simulink model "inga2s"  (R2013a)
settings: Solver=ode45  StartTime=0.0  StopTime=100.0  RelTol=1e-3
values from neighbouring files (symbols this model uses):
  b = 0.3    [Inga.m]
  g = 9.81    [Inga.m]
  J = 0.008    [Inga.m]
  l = 6    [Inga.m]
  m = 0.4    [Inga.m]
  M = 0.6    [Inga.m]
settings Model: Creator=Kinga  LastModifiedBy=rudi
settings DataIOCC: SignalLoggingSaveFormat=ModelDataLogs
settings DebuggingCC: UnderspecifiedInitializationDetection=Simplified  MultiTaskDSMMsg=warning  MultiTaskCondExecSysMsg=none  StateNameClashWarn=none  StrictBusMsg=ErrorOnBusTreatedAsVector  NonBusSignalsTreatedAsBus=error
settings RTWCC: IncludeERTFirstTime=on
settings GRTTargetCC: CodeReplacementLibrary=None  CPPClassGenCompliant=on

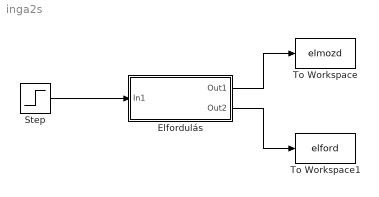
== system inga2s ==
  Elfordulás : Subsystem
  Step : Step  SampleTime=0
  To Workspace : ToWorkspace  VariableName=elmozd  SampleTime=-1  SaveFormat=Timeseries
  To Workspace1 : ToWorkspace  VariableName=elford  SampleTime=-1  SaveFormat=Timeseries
  wires:
  Elfordulás/1(Out1) -> To Workspace/1
  Elfordulás/2(Out2) -> To Workspace1/1
  Step/1 -> Elfordulás/1(In1)

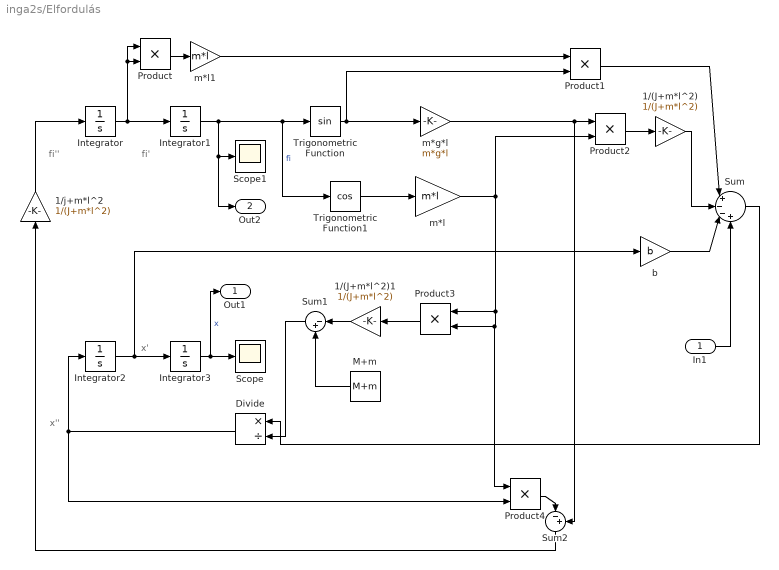
== system inga2s/Elfordulás ==
  note: x''
  note: x'
  note: fi''
  note: fi'
  In1 : Inport
  1/(J+m*l^2) : Gain  Gain=1/(J+m*l^2)
  1/(J+m*l^2)1 : Gain  Gain=1/(J+m*l^2)
  1/j+m*l^2 : Gain  Gain=1/(J+m*l^2)
  Divide : Product  Inputs=*/
  Integrator{,1..3} (4 alike) : Integrator
  M+m : Constant  Value=M+m
  Product{,1..4} (5 alike) : Product
  Scope : Scope
      settings: SaveName=ScopeData2
  Scope1 : Scope
      settings: SaveName=ScopeData3
  Sum : Sum  Inputs=|+--+
  Sum1 : Sum  Inputs=|-+
  Sum2 : Sum  Inputs=|-+
  Trigonometric Function : Trigonometry
  Trigonometric Function1 : Trigonometry  Operator=cos
  b : Gain  Gain=b
  m*g*l : Gain  Gain=m*g*l
  m*l : Gain  Gain=m*l
  m*l1 : Gain  Gain=m*l
  Out1 : Outport
  Out2 : Outport  Port=2
  wires:
  Integrator/1 -> Integrator1/1, Product/1, Product/2
  Integrator2/1 -> b/1, Integrator3/1
  Integrator1/1 -> Trigonometric Function1/1, Trigonometric Function/1, Out2/1, Scope1/1  "fi"
  Trigonometric Function/1 -> Product1/2, m*g*l/1
  Trigonometric Function1/1 -> m*l/1
  Product/1 -> m*l1/1
  m*l1/1 -> Product1/1
  m*g*l/1 -> Sum2/2, Product2/1
  m*l/1 -> Product3/1, Product3/2, Product4/1, Product2/2
  Product2/1 -> 1/(J+m*l^2)/1
  Product1/1 -> Sum/1
  1/(J+m*l^2)/1 -> Sum/2
  b/1 -> Sum/3
  Product3/1 -> 1/(J+m*l^2)1/1
  1/(J+m*l^2)1/1 -> Sum1/1
  Divide/1 -> Product4/2, Integrator2/1
  1/j+m*l^2/1 -> Integrator/1
  Product4/1 -> Sum2/1
  Sum2/1 -> 1/j+m*l^2/1
  Integrator3/1 -> Out1/1, Scope/1  "x"
  Sum1/1 -> Divide/2
  Sum/1 -> Divide/1
  In1/1 -> Sum/4
  M+m/1 -> Sum1/2
